simulink model "DoF6"  (Simulink 7.3)
settings: Solver=ode4  StartTime=0.0  StopTime=10.0  FixedStep=0.1  RelTol=1e-3
undefined symbols (not defined in the file): e0_0, e1_0, e2_0, e3_0
libraries: simulink x6, aerolibtransform2 x3, aerolibutil x1, aerolibanim x1
settings Model: Creator=WangHua  LastModifiedBy=WangHua

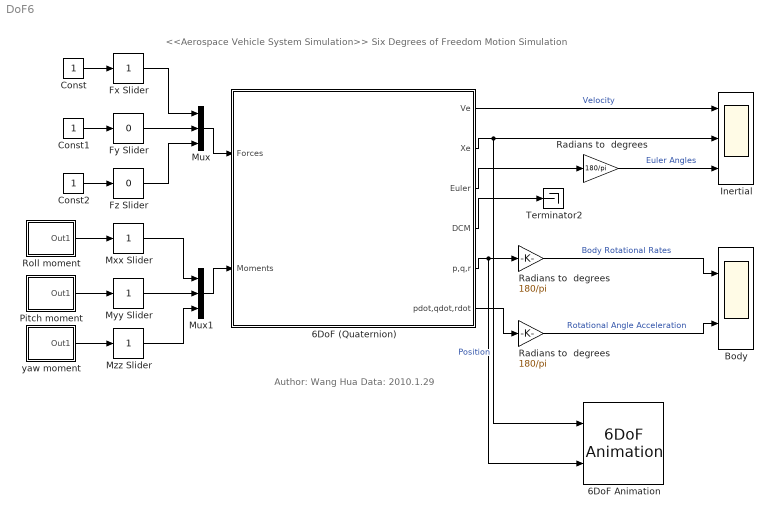
== system DoF6 ==
  note: <<Aerospace Vehicle System Simulation>>
      | Six Degrees of Freedom Motion Simulation
  note: Author: Wang Hua
      | Data: 2010.1.29
  6DoF (Quaternion) : Subsystem  mask{xme_0=[0 0 0], Vme_0=[0 0 0], eul_0=[0 0 0], pm_0=[0 0 0], mass_0=1.0, inertia=eye(3).*10, k_quat=1.0}
      mask prompts: xme_0 "Initial position in inertial axes [Xe,Ye,Ze]:"; Vme_0 "Initial velocity in inertial axes [U,v,w]:"; eul_0 "Initial Euler orientation [yaw, pitch, roll](321 sequence):"; pm_0 "Initial body rotation rates [p,q,r]:"; mass_0 "Initial mass:"; k_quat "Gain for quaternion normalization:"
      mask help: Integrate the six-degrees-of-freedom equations of motion.
  6DoF Animation : aerolibanim/6DoF Animation  SystemSampleTime=-1  u1=[0 40 0 40 0 40]  u2=0.1  u3=10  u4=[0 100 0]  u5=Fly alongside  u6=[10 10 50]  u7=45  u8=on
  Body : Scope  NumInputPorts=2
      settings: TimeRange=10  YMin=-10~-10  YMax=10~10
  Const : Constant  OutDataType=sfix(16)  OutScaling=2^0
  Const1 : Constant  OutDataType=sfix(16)  OutScaling=2^0
  Const2 : Constant  OutDataType=sfix(16)  OutScaling=2^0
  Fx Slider : simulink/Math Operations/Slider Gain  SystemSampleTime=-1  low=-1  gain=1  high=1
  Fy Slider : simulink/Math Operations/Slider Gain  SystemSampleTime=-1  low=-1  gain=0  high=1
  Fz Slider : simulink/Math Operations/Slider Gain  SystemSampleTime=-1  low=-1  gain=0  high=1
  Inertial : Scope  NumInputPorts=3
      settings: TickLabels=on  TimeRange=10  YMin=-2~-10~-50  YMax=6~40~100  SaveName=InertialData
  Mux : Mux  Inputs=3
  Mux1 : Mux  Inputs=3
  Mxx Slider : simulink/Math Operations/Slider Gain  SystemSampleTime=-1  low=-5  gain=1  high=10
  Myy Slider : simulink/Math Operations/Slider Gain  SystemSampleTime=-1  low=-10  gain=1  high=10
  Mzz Slider : simulink/Math Operations/Slider Gain  SystemSampleTime=-1  low=-1  gain=1  high=1
  Pitch moment : Subsystem  mask(timed input){t=[0 3 3.1 4 4.1 5 5.1  7.5 7.6 8.5 8.6 9.5 9.6 10], u=[0 0  1 1 -1 -1.005 0 0 -1 -1 1 1 0 0]*3.138/2}
      mask prompts: t "time values:"; u "input values"
      mask Display: plot(t,u)
  Radians to  degrees : Gain  Gain=180/pi  ParameterDataType=sfix(16)  ParameterScaling=2^0  OutDataType=sfix(16)  OutScaling=2^0  SaturateOnIntegerOverflow=on  OutDataTypeStr=Inherit: Same as input  ParamDataTypeStr=Inherit: Same as input
  "Radians to  degrees " : Gain  Gain=180/pi  ParameterDataType=sfix(16)  ParameterScaling=2^0  OutDataType=sfix(16)  OutScaling=2^0  SaturateOnIntegerOverflow=on  OutDataTypeStr=Inherit: Same as input  ParamDataTypeStr=Inherit: Same as input
  "Radians to  degrees  " : Gain  Gain=180/pi  ParameterDataType=sfix(16)  ParameterScaling=2^0  OutDataType=sfix(16)  OutScaling=2^0  SaturateOnIntegerOverflow=on  OutDataTypeStr=Inherit: Same as input  ParamDataTypeStr=Inherit: Same as input
  Roll moment : Subsystem  mask(timed input){t=[0 1 1.1 2 2.1  10], u=[1 1 -1 -.998  0 0]*3.144/2}
      mask prompts: t "time values:"; u "input values"
      mask Display: plot(t,u)
  Terminator2 : Terminator
  yaw moment : Subsystem  mask(timed input){t=[0 6 6.1 7 7.1 8 8.1 10], u=[0 0  -1 -1 1 1 0 0]*3.1/2}
      mask prompts: t "time values:"; u "input values"
      mask Display: plot(t,u)
  wires:
  yaw moment/1(Out1) -> Mzz Slider/1
  Pitch moment/1(Out1) -> Myy Slider/1
  Roll moment/1(Out1) -> Mxx Slider/1
  Const2/1 -> Fz Slider/1
  Const1/1 -> Fy Slider/1
  Const/1 -> Fx Slider/1
  Mux1/1 -> 6DoF (Quaternion)/2(Moments)
  Mzz Slider/1 -> Mux1/3
  Myy Slider/1 -> Mux1/2
  Mxx Slider/1 -> Mux1/1
  Mux/1 -> 6DoF (Quaternion)/1(Forces)
  Fy Slider/1 -> Mux/2
  Fz Slider/1 -> Mux/3
  Fx Slider/1 -> Mux/1
  Radians to  degrees/1 -> Inertial/3  "Euler Angles"
  6DoF (Quaternion)/1(Ve) -> Inertial/1  "Velocity"
  6DoF (Quaternion)/2(Xe) -> Inertial/2, 6DoF Animation/1  "Position"
  6DoF (Quaternion)/3(Euler) -> Radians to  degrees/1
  6DoF (Quaternion)/4(DCM) -> Terminator2/1
  6DoF (Quaternion)/5(p,q,r) -> "Radians to  degrees "/1, 6DoF Animation/2
  6DoF (Quaternion)/6(pdot,qdot,rdot) -> "Radians to  degrees  "/1
  "Radians to  degrees "/1 -> Body/1  "Body Rotational Rates"
  "Radians to  degrees  "/1 -> Body/2  "Rotational Angle Acceleration"

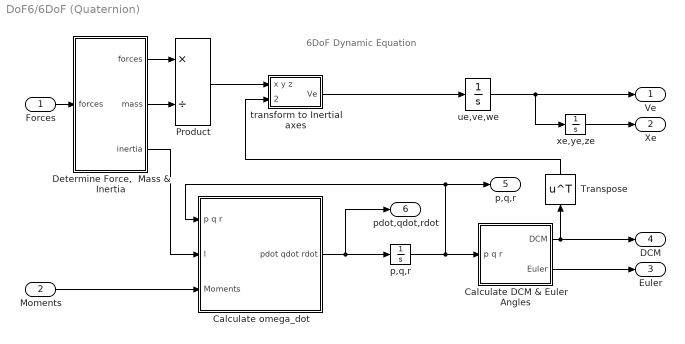
== system DoF6/6DoF (Quaternion) ==
  note: 6DoF Dynamic Equation
  Forces : Inport  OutDataType=sfix(16)  OutScaling=2^0
  Moments : Inport  Port=2  OutDataType=sfix(16)  OutScaling=2^0
  Calculate DCM & Euler Angles : Subsystem  AncestorBlock=aerolib6dofsys/DCM & Euler Angles (Quaternion)
      mask Type: DCM & Euler Angles (Quaternion)
  Calculate omega_dot : Subsystem
  "Determine Force,  Mass & Inertia" : Subsystem
      mask Type: Mass & Inertia (fixed)
  Product : Product  Inputs=*/  OutDataType=sfix(16)  OutScaling=2^0  SaturateOnIntegerOverflow=on  OutDataTypeStr=Inherit: Same as first input
  Transpose : Math  Operator=transpose  OutDataType=sfix(16)  OutScaling=2^0  SaturateOnIntegerOverflow=on
  "p,q,r " : Integrator  InitialCondition=pm_0
  "transform to Inertial axes " : Subsystem
      mask Type: Vector Transformation
      mask Display: disp('L_EB')
  ue,ve,we : Integrator  InitialCondition=Vme_0
  xe,ye,ze : Integrator  InitialCondition=xme_0
  Ve : Outport  OutDataType=sfix(16)  OutScaling=2^0
  Xe : Outport  Port=2  OutDataType=sfix(16)  OutScaling=2^0
  Euler : Outport  Port=3  OutDataType=sfix(16)  OutScaling=2^0
  DCM : Outport  Port=4  OutDataType=sfix(16)  OutScaling=2^0
  p,q,r : Outport  Port=5  OutDataType=sfix(16)  OutScaling=2^0
  pdot,qdot,rdot : Outport  Port=6  OutDataType=sfix(16)  OutScaling=2^0
  wires:
  "Determine Force,  Mass & Inertia"/3(inertia) -> Calculate omega_dot/2(I)
  Calculate DCM & Euler Angles/2(Euler) -> Euler/1
  xe,ye,ze/1 -> Xe/1
  "p,q,r "/1 -> Calculate DCM & Euler Angles/1(p q r), Calculate omega_dot/1(p q r), p,q,r/1
  Moments/1 -> Calculate omega_dot/3(Moments)
  Forces/1 -> "Determine Force,  Mass & Inertia"/1(forces)
  Product/1 -> "transform to Inertial axes "/1(x y z)
  Calculate DCM & Euler Angles/1(DCM) -> Transpose/1, DCM/1
  Transpose/1 -> "transform to Inertial axes "/2(transform coefficients)
  "Determine Force,  Mass & Inertia"/2(mass) -> Product/2
  Calculate omega_dot/1(pdot qdot rdot) -> pdot,qdot,rdot/1, "p,q,r "/1
  "Determine Force,  Mass & Inertia"/1("forces ") -> Product/1
  "transform to Inertial axes "/1(Ve) -> ue,ve,we/1
  ue,ve,we/1 -> xe,ye,ze/1, Ve/1

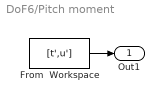
== system DoF6/Pitch moment ==
  From  Workspace : FromWorkspace  VariableName=[t',u']  SampleTime=0
  Out1 : Outport  OutDataType=sfix(16)  OutScaling=2^0  InitialOutput=0
  wires:
  From  Workspace/1 -> Out1/1

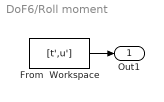
== system DoF6/Roll moment ==
  From  Workspace : FromWorkspace  VariableName=[t',u']  SampleTime=0
  Out1 : Outport  OutDataType=sfix(16)  OutScaling=2^0  InitialOutput=0
  wires:
  From  Workspace/1 -> Out1/1

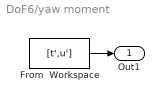
== system DoF6/yaw moment ==
  From  Workspace : FromWorkspace  VariableName=[t',u']  SampleTime=0
  Out1 : Outport  OutDataType=sfix(16)  OutScaling=2^0  InitialOutput=0
  wires:
  From  Workspace/1 -> Out1/1

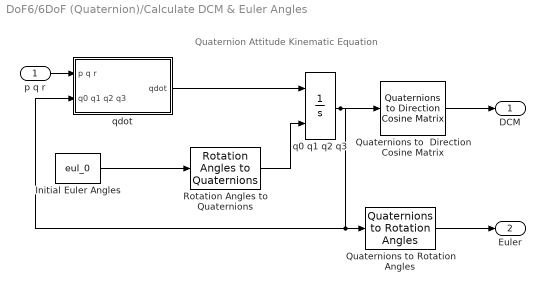
== system DoF6/6DoF (Quaternion)/Calculate DCM & Euler Angles ==
  note: Quaternion Attitude Kinematic Equation
  p q r : Inport  OutDataType=sfix(16)  OutScaling=2^0
  Initial Euler Angles : Constant  Value=eul_0  OutDataType=sfix(16)  OutScaling=2^0
  Quaternions to  Direction Cosine Matrix : aerolibtransform2/Quaternions to  Direction Cosine Matrix  SystemSampleTime=-1
  Quaternions to Rotation Angles : aerolibtransform2/Quaternions to Rotation Angles  SystemSampleTime=-1  rotationOrder=ZYX
  Rotation Angles to Quaternions : aerolibtransform2/Rotation Angles to Quaternions  SystemSampleTime=-1  rotationOrder=ZYX
  q0 q1 q2 q3 : Integrator  InitialConditionSource=external  InitialCondition=[e0_0 e1_0 e2_0 e3_0]
  qdot : Subsystem
  DCM : Outport  OutDataType=sfix(16)  OutScaling=2^0
  Euler : Outport  Port=2  OutDataType=sfix(16)  OutScaling=2^0
  wires:
  qdot/1(qdot) -> q0 q1 q2 q3/1
  q0 q1 q2 q3/1 -> qdot/2(q0 q1 q2 q3), Quaternions to Rotation Angles/1, Quaternions to  Direction Cosine Matrix/1
  Rotation Angles to Quaternions/1 -> q0 q1 q2 q3/2
  Initial Euler Angles/1 -> Rotation Angles to Quaternions/1
  p q r/1 -> qdot/1(p q r)
  Quaternions to  Direction Cosine Matrix/1 -> DCM/1
  Quaternions to Rotation Angles/1 -> Euler/1

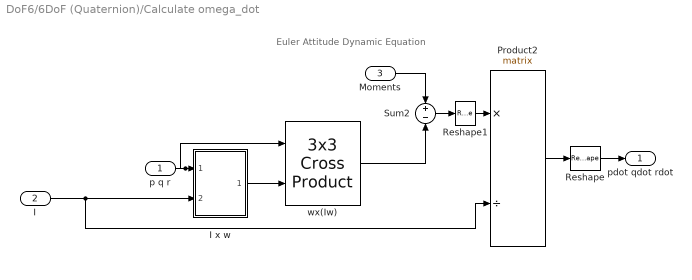
== system DoF6/6DoF (Quaternion)/Calculate omega_dot ==
  note: Euler Attitude Dynamic Equation
  p q r : Inport  OutDataType=sfix(16)  OutScaling=2^0
  I : Inport  Port=2  OutDataType=sfix(16)  OutScaling=2^0
  Moments : Inport  Port=3  OutDataType=sfix(16)  OutScaling=2^0
  I x w : Subsystem
  Product2 : Product  Inputs=*/  Multiplication=Matrix(*)  OutDataType=sfix(16)  OutScaling=2^0  SaturateOnIntegerOverflow=on  OutDataTypeStr=Inherit: Same as first input
  Reshape : Reshape
  Reshape1 : Reshape  OutputDimensionality=Row vector (2-D)
  Sum2 : Sum  Inputs=+-  OutDataType=sfix(16)  OutScaling=2^0  SaturateOnIntegerOverflow=on
  wx(Iw) : aerolibutil/3x3 Cross Product  SystemSampleTime=-1
  pdot qdot rdot : Outport  OutDataType=sfix(16)  OutScaling=2^0
  wires:
  Reshape1/1 -> Product2/1
  I x w/1(I * w) -> wx(Iw)/2
  wx(Iw)/1 -> Sum2/2
  Moments/1 -> Sum2/1
  Sum2/1 -> Reshape1/1
  Product2/1 -> Reshape/1
  p q r/1 -> wx(Iw)/1, I x w/1(p q r)
  I/1 -> I x w/2(Inertia), Product2/2
  Reshape/1 -> pdot qdot rdot/1

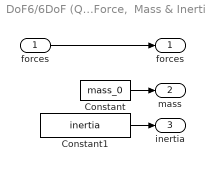
== system DoF6/6DoF (Quaternion)/Determine Force,  Mass & Inertia ==
  forces : Inport  OutDataType=sfix(16)  OutScaling=2^0
  Constant : Constant  Value=mass_0  OutDataType=sfix(16)  OutScaling=2^0  OutDataTypeStr=Inherit: Inherit via back propagation
  Constant1 : Constant  Value=inertia  OutDataType=sfix(16)  OutScaling=2^0  OutDataTypeStr=Inherit: Inherit via back propagation
  "forces " : Outport  OutDataType=sfix(16)  OutScaling=2^0
  mass : Outport  Port=2  OutDataType=sfix(16)  OutScaling=2^0
  inertia : Outport  Port=3  OutDataType=sfix(16)  OutScaling=2^0
  wires:
  Constant/1 -> mass/1
  Constant1/1 -> inertia/1
  forces/1 -> "forces "/1

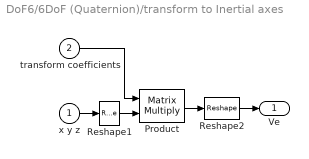
== system DoF6/6DoF (Quaternion)/transform to Inertial axes  ==
  x y z : Inport  OutDataType=sfix(16)  OutScaling=2^0
  transform coefficients : Inport  Port=2  OutDataType=sfix(16)  OutScaling=2^0
  Product : Product  Multiplication=Matrix(*)  OutDataType=sfix(16)  OutScaling=2^0  SaturateOnIntegerOverflow=on  InputSameDT=on  OutDataTypeStr=Inherit: Same as first input
  Reshape1 : Reshape  OutputDimensionality=Column vector (2-D)
  Reshape2 : Reshape
  Ve : Outport  OutDataType=sfix(16)  OutScaling=2^0
  wires:
  Product/1 -> Reshape2/1
  transform coefficients/1 -> Product/1
  x y z/1 -> Reshape1/1
  Reshape1/1 -> Product/2
  Reshape2/1 -> Ve/1

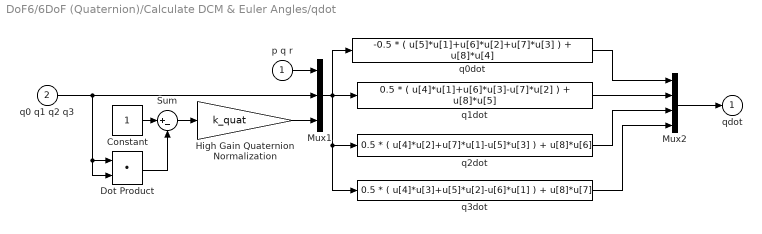
== system DoF6/6DoF (Quaternion)/Calculate DCM & Euler Angles/qdot ==
  p q r : Inport  OutDataType=sfix(16)  OutScaling=2^0
  q0 q1 q2 q3 : Inport  Port=2  OutDataType=sfix(16)  OutScaling=2^0
  Constant : Constant  OutDataType=sfix(16)  OutScaling=2^0
  Dot Product : DotProduct  OutDataType=sfix(16)  OutScaling=2^-10  OutDataTypeStr=Inherit: Inherit via internal rule
  High Gain Quaternion Normalization : Gain  Gain=k_quat  ParameterDataType=sfix(16)  ParameterScaling=2^0  OutDataType=sfix(16)  OutScaling=2^0  SaturateOnIntegerOverflow=on  OutDataTypeStr=Inherit: Same as input  ParamDataTypeStr=Inherit: Same as input
  Mux1 : Mux  Inputs=[3 4 1]
  Mux2 : Mux
  Sum : Sum  Inputs=|+-  OutDataType=sfix(16)  OutScaling=2^0  SaturateOnIntegerOverflow=on  InputSameDT=on  OutDataTypeStr=Inherit: Same as first input
  q0dot : Fcn  Expr=-0.5 * ( u[5]*u[1]+u[6]*u[2]+u[7]*u[3] ) + u[8]*u[4]
  q1dot : Fcn  Expr=0.5 * ( u[4]*u[1]+u[6]*u[3]-u[7]*u[2] ) + u[8]*u[5]
  q2dot : Fcn  Expr=0.5 * ( u[4]*u[2]+u[7]*u[1]-u[5]*u[3] ) + u[8]*u[6]
  q3dot : Fcn  Expr=0.5 * ( u[4]*u[3]+u[5]*u[2]-u[6]*u[1] ) + u[8]*u[7]
  qdot : Outport  OutDataType=sfix(16)  OutScaling=2^0  InitialOutput=0
  wires:
  q0 q1 q2 q3/1 -> Mux1/2, Dot Product/2, Dot Product/1
  q3dot/1 -> Mux2/4
  Mux1/1 -> q1dot/1, q0dot/1, q3dot/1, q2dot/1
  q2dot/1 -> Mux2/3
  q1dot/1 -> Mux2/2
  q0dot/1 -> Mux2/1
  Mux2/1 -> qdot/1
  Constant/1 -> Sum/1
  Sum/1 -> High Gain Quaternion Normalization/1
  High Gain Quaternion Normalization/1 -> Mux1/3
  Dot Product/1 -> Sum/2
  p q r/1 -> Mux1/1

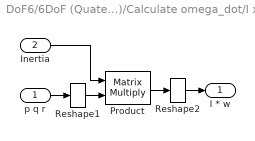
== system DoF6/6DoF (Quaternion)/Calculate omega_dot/I x w ==
  p q r : Inport  OutDataType=sfix(16)  OutScaling=2^0
  Inertia : Inport  Port=2  OutDataType=sfix(16)  OutScaling=2^0
  Product : Product  Multiplication=Matrix(*)  OutDataType=sfix(16)  OutScaling=2^0  SaturateOnIntegerOverflow=on  InputSameDT=on  OutDataTypeStr=Inherit: Same as first input
  Reshape1 : Reshape  OutputDimensionality=Column vector (2-D)
  Reshape2 : Reshape
  I * w : Outport  OutDataType=sfix(16)  OutScaling=2^0
  wires:
  Reshape2/1 -> I * w/1
  Reshape1/1 -> Product/2
  p q r/1 -> Reshape1/1
  Inertia/1 -> Product/1
  Product/1 -> Reshape2/1
